simulink model "Pan"  (Simulink 6.1)
settings: Solver=ode45  StartTime=0.0  StopTime=20  RelTol=1e-3
values from neighbouring files (symbols this model uses):
  delayImageProc = .095    (= 0.095)    [simPan.m]    (also in simZoom.m = 0.1)
  delayInquiryPan = .015    (= 0.015)    [simPan.m]
  gainPixelsPerDegree = 4    [simPan.m]
  periodPanControl = periodFrame * framesPerPan    (= 0.066)    [simPan.m]
  pPan = 1/(1+s/15)^2    [simPan.m]
  rateLimitPan = 290    [simPan.m]
settings Model: LastModifiedBy=Big E
settings DebuggingCC: SolverPrmCheckMsg=warning

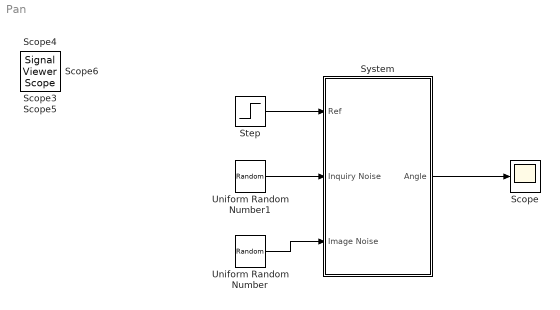
== system Pan ==
  Scope : Scope
  Step : Step  After=120  SampleTime=0
  System : Subsystem
  Uniform Random Number : UniformRandomNumber  Minimum=-0.5  Maximum=0.5  SampleTime=0
  Uniform Random Number1 : UniformRandomNumber  Minimum=-0.07  Maximum=0.07  SampleTime=0
  Scope{3..6} (4 alike) : SignalViewerScope  IOType=viewer  RefreshTime=0.035000
  wires:
  Step/1 -> System/1(Ref)
  System/1(Angle) -> Scope/1
  Uniform Random Number/1 -> System/3(Image Noise)
  Uniform Random Number1/1 -> System/2(Inquiry Noise)

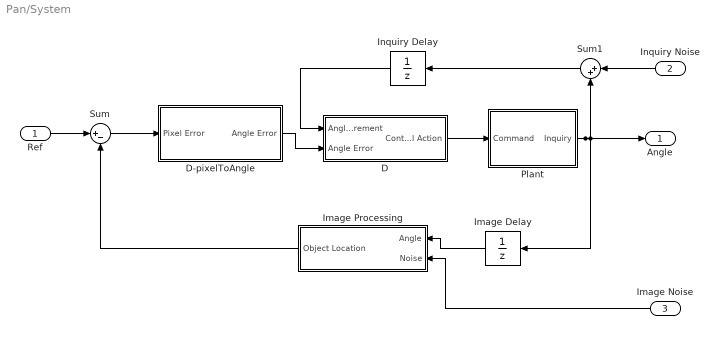
== system Pan/System ==
  Ref : Inport  Port=1  LatchInput=off
  Inquiry Noise : Inport  Orientation=left  Port=2  LatchInput=off
  Image Noise : Inport  Orientation=left  Port=3  LatchInput=off
  D : Subsystem
  D-pixelToAngle : Subsystem
  Image Delay : UnitDelay  Orientation=left  SampleTime=delayImageProc
  Image Processing : Subsystem  Orientation=left
  Inquiry Delay : UnitDelay  Orientation=left  SampleTime=delayInquiryPan
  Plant : Subsystem
  Sum : Sum  Inputs=|+-
  Sum1 : Sum  Orientation=left  Inputs=|++
  Angle : Outport
  wires:
  Plant/1(Inquiry) -> Angle/1, Sum1/2, Image Delay/1
  Ref/1 -> Sum/1
  Sum/1 -> D-pixelToAngle/1(Pixel Error)
  D/1(Control Action) -> Plant/1(Command)
  D-pixelToAngle/1(Angle Error) -> D/2(Angle Error)
  Inquiry Delay/1 -> D/1(Angle Measurement)
  Sum1/1 -> Inquiry Delay/1
  Inquiry Noise/1 -> Sum1/1
  Image Noise/1 -> Image Processing/2(Noise)
  Image Delay/1 -> Image Processing/1(Angle)
  Image Processing/1(Object Location) -> Sum/2

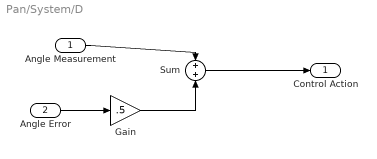
== system Pan/System/D ==
  Angle Measurement : Inport  Port=1  LatchInput=off
  Angle Error : Inport  Port=2  LatchInput=off
  Gain : Gain  Gain=.5
  Sum : Sum  Inputs=+|+
  Control Action : Outport
  wires:
  Angle Measurement/1 -> Sum/1
  Sum/1 -> Control Action/1
  Angle Error/1 -> Gain/1
  Gain/1 -> Sum/2

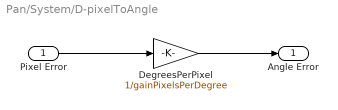
== system Pan/System/D-pixelToAngle ==
  Pixel Error : Inport  Port=1  LatchInput=off
  DegreesPerPixel : Gain  Gain=1/gainPixelsPerDegree
  Angle Error : Outport
  wires:
  Pixel Error/1 -> DegreesPerPixel/1
  DegreesPerPixel/1 -> Angle Error/1

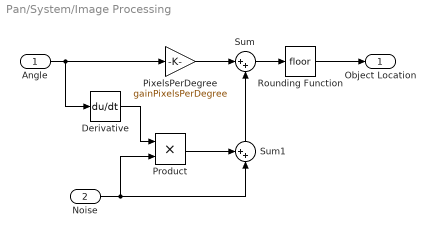
== system Pan/System/Image Processing ==
  Angle : Inport  Port=1  LatchInput=off
  Noise : Inport  Port=2  LatchInput=off
  Derivative : Derivative
  PixelsPerDegree : Gain  Gain=gainPixelsPerDegree
  Product : Product  RndMeth=Zero
  Rounding Function : Rounding
  Sum : Sum  Inputs=|++
  Sum1 : Sum  Orientation=up  Inputs=++|
  Object Location : Outport
  wires:
  Angle/1 -> PixelsPerDegree/1, Derivative/1
  Rounding Function/1 -> Object Location/1
  PixelsPerDegree/1 -> Sum/1
  Sum/1 -> Rounding Function/1
  Sum1/1 -> Sum/2
  Noise/1 -> Product/2, Sum1/2
  Derivative/1 -> Product/1
  Product/1 -> Sum1/1

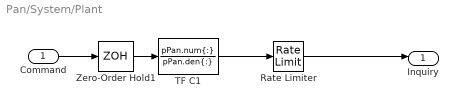
== system Pan/System/Plant ==
  Command : Inport  Port=1  LatchInput=off
  Rate Limiter : RateLimiter  RisingSlewLimit=rateLimitPan  FallingSlewLimit=-rateLimitPan  SampleTimeMode=inherited
  TF C1 : TransferFcn  Numerator=pPan.num{:}  Denominator=pPan.den{:}
  Zero-Order Hold1 : ZeroOrderHold  SampleTime=periodPanControl
  Inquiry : Outport
  wires:
  Command/1 -> Zero-Order Hold1/1
  Zero-Order Hold1/1 -> TF C1/1
  Rate Limiter/1 -> Inquiry/1
  TF C1/1 -> Rate Limiter/1
